simulink model "EarlyReturn15_2018a"  (R2018a)
settings: Solver=VariableStepAuto  StartTime=0.0  StopTime=0.1  RelTol=1e-3
settings Model: Creator=BEAR  LastModifiedBy=apple

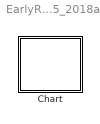
== system EarlyReturn15_2018a ==
  Chart : Stateflow chart  TreatAsAtomicUnit=on

== stateflow chart EarlyReturn15_2018a/Chart ==
  state S
    en: fprintf("enS")
    state A1 [parallel]
      en: fprintf("enA1")
      settings: executionOrder=1
      state A1a
        en: fprintf("enA1a")
      state A1b
        en: fprintf("enA1b")
      (default) -> A1a
      A1a -> A1b : {fprintf("ca")}/{E;fprintf("ta")}
    state A2 [parallel]
      en: fprintf("enA2")
      settings: executionOrder=2
  state B
    en: fprintf("enB")
  (default) -> S
  S -> B : E
  events: E local FUNCTION_CALL_EVENT
